simulink model "Act2_espacio_estados"  (R2024a)
settings: Solver=VariableStepAuto  StartTime=0.0  StopTime=100  RelTol=1e-3

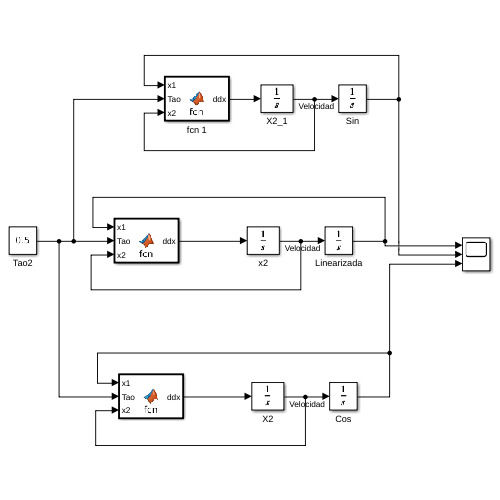
[thumbnail: Simulink's stored preview of the top-level diagram]
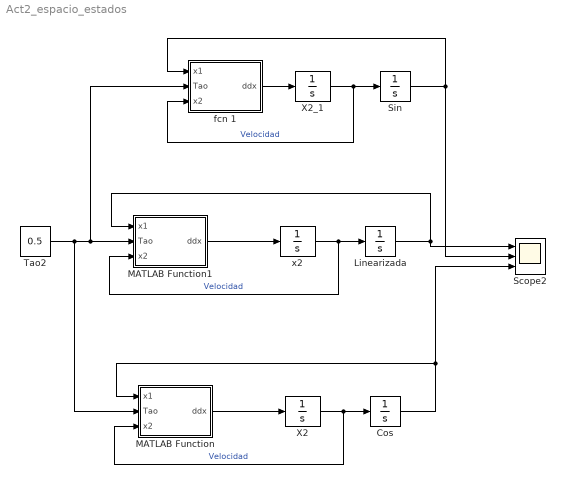
== system Act2_espacio_estados ==
  Cos : Integrator  InitialCondition=2*pi
  Linearizada : Integrator  InitialCondition=2*pi
  MATLAB Function : MATLAB Function  TreatAsAtomicUnit=on
  MATLAB Function1 : MATLAB Function  TreatAsAtomicUnit=on
  Scope2 : Scope  NumInputPorts=3
  Sin : Integrator  InitialCondition=2*pi
  Tao2 : Constant  Value=0.5
  X2 : Integrator
  X2_1 : Integrator
  fcn 1 : MATLAB Function  TreatAsAtomicUnit=on
  x2 : Integrator
  wires:
  X2/1 -> MATLAB Function/3(x2), Cos/1  "Velocidad"
  Cos/1 -> Scope2/3, MATLAB Function/1(x1)
  Tao2/1 -> MATLAB Function/2(Tao), fcn 1/2(Tao), MATLAB Function1/2(Tao)
  X2_1/1 -> fcn 1/3(x2), Sin/1  "Velocidad"
  fcn 1/1(ddx) -> X2_1/1
  Sin/1 -> Scope2/2, fcn 1/1(x1)
  MATLAB Function/1(ddx) -> X2/1
  MATLAB Function1/1(ddx) -> x2/1
  x2/1 -> MATLAB Function1/3(x2), Linearizada/1  "Velocidad"
  Linearizada/1 -> MATLAB Function1/1(x1), Scope2/1

== matlab function Act2_espacio_estados/MATLAB Function ==
  data: x1 input; Tao input; x2 input; ddx output
function ddx = fcn(x1,Tao, x2)

k = 0.01;
m = 0.75;
l = 0.36;
g = 9.8;

%Arguments calculation
a= l/2;
J = 4/3*m*a*a;

ddx=Tao/J - k*x2/J -m*g*a*cos(x1)/J;
end

== matlab function Act2_espacio_estados/fcn 1 ==
  data: x1 input; Tao input; x2 input; ddx output
function ddx = fcn(x1,Tao, x2)

k = 0.01;
m = 0.75;
l = 0.36;
g = 9.8;

%Arguments calculation
a= l/2;
J = 4/3*m*a*a;

ddx=Tao/J - k*x2/J -m*g*a*sin(x1)/J;
end

== matlab function Act2_espacio_estados/MATLAB Function1 ==
  data: x1 input; Tao input; x2 input; ddx output
function ddx = fcn(x1,Tao, x2)

k = 0.01;
m = 0.75;
l = 0.36;
g = 9.8;

%Arguments calculation
a= l/2;
J = 4/3*m*a*a;

ddx=Tao/J - k*x2/J -m*g*a*x1/J;
end
